simulink model "full_system_nios"  (R2021b)
settings: Solver=FixedStepDiscrete  StartTime=0.0  StopTime=250000  RelTol=1e-3
model workspace (MAT data in the model file):
  out_size = 0
undefined symbols (not defined in the file): betas, bias, DiscIntNeverNeededParam, mus, scale, sigmas
libraries: hdlsllib x2
(part 1 of 3)
settings Model: DataTypeOverride=Off  SimulationMode=accelerator  Creator=local_adm  LastModifiedBy=local_adm
settings SolverCC: AlgebraicLoopSolver=TrustRegion
settings DataIOCC: LimitDataPoints=on  SaveOutput=off  SaveTime=off
settings OptimizationCC: BlockReduction=off  ConditionallyExecuteInputs=off  DefaultParameterBehavior=Inlined  LifeSpan=inf
settings DebuggingCC: AlgebraicLoopMsg=error  SingleTaskRateTransMsg=error  ParameterPrecisionLossMsg=none  AllowSymbolicDim=off  StrictBusMsg=ErrorOnBusTreatedAsVector  SFUnexpectedBacktrackingDiag=warning  SFNoUnconditionalDefaultTransitionDiag=warning  SFExecutionAtInitializationDiag=none  SFMachineParentedDataDiag=warning  ArithmeticOperatorsInVariantConditions=warning
settings HardwareCC: ProdBitPerPointer=32  ProdBitPerSizeT=32  ProdBitPerPtrDiffT=32  ProdLargestAtomicFloat=None  ProdIntDivRoundTo=Undefined  ProdEndianess=Unspecified  ProdWordSize=32  ProdHWDeviceType=ASIC/FPGA->ASIC/FPGA  ProdEqTarget=off
settings SFSimCC: SimUseLocalCustomCode=off  CustomCodeUndefinedFunction=UseInterfaceOnly
settings RTWCC: RTWUseLocalCustomCode=off
settings CodeAppCC: StateflowObjectComments=on
settings GRTTargetCC: TargetLangStandard=C89/C90 (ANSI)
settings ConfigComp: CovScope=ReferencedModels  CovMetricSettings=dw  CovSaveCumulativeToWorkspaceVar=on  CovSaveSingleToWorkspaceVar=on  CovExternalEMLEnable=off  CovSFcnEnable=off

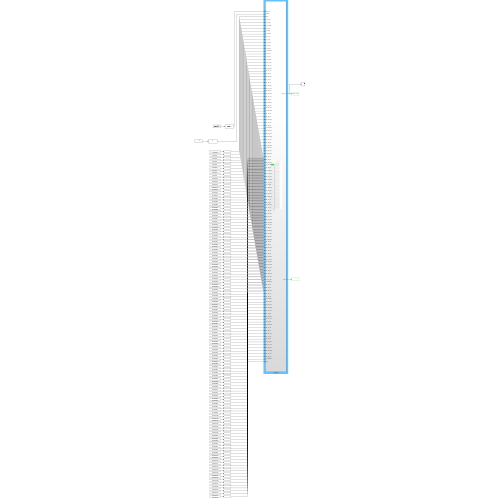
[thumbnail: Simulink's stored preview of the top-level diagram]
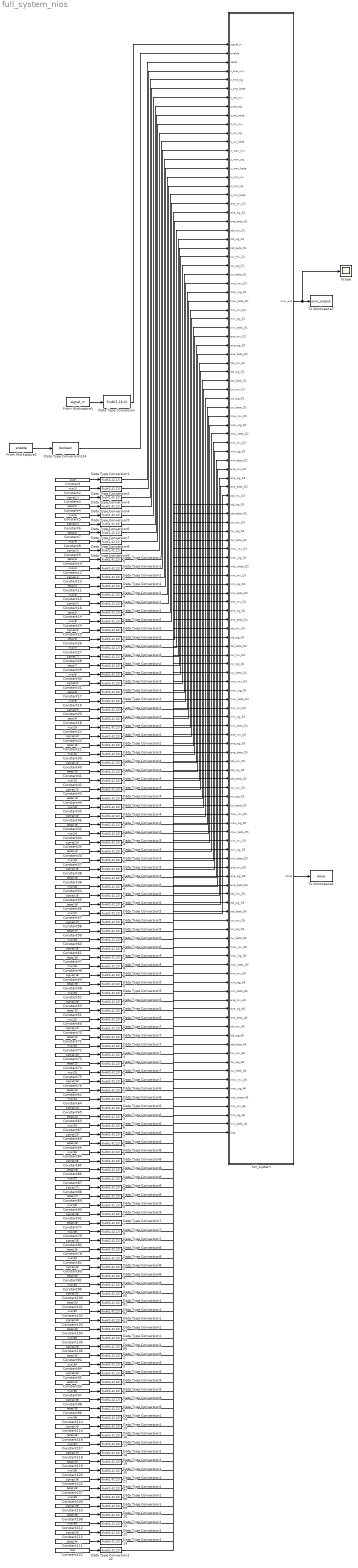
== system full_system_nios ==
  Constant : Constant  Value=scale  VectorParams1D=off  SampleTime=-1
  Constant10 : Constant  Value=betas(3)  VectorParams1D=off  SampleTime=-1
  Constant100 : Constant  Value=sigmas(31)  VectorParams1D=off  SampleTime=-1
  Constant101 : Constant  Value=betas(31)  VectorParams1D=off  SampleTime=-1
  Constant102 : Constant  Value=mus(32)  VectorParams1D=off  SampleTime=-1
  Constant103 : Constant  Value=sigmas(32)  VectorParams1D=off  SampleTime=-1
  Constant104 : Constant  Value=betas(32)  VectorParams1D=off  SampleTime=-1
  Constant105 : Constant  Value=mus(33)  VectorParams1D=off  SampleTime=-1
  Constant106 : Constant  Value=sigmas(33)  VectorParams1D=off  SampleTime=-1
  Constant107 : Constant  Value=betas(38)  VectorParams1D=off  SampleTime=-1
  Constant108 : Constant  Value=betas(39)  VectorParams1D=off  SampleTime=-1
  Constant109 : Constant  Value=mus(39)  VectorParams1D=off  SampleTime=-1
  Constant11 : Constant  Value=betas(4)  VectorParams1D=off  SampleTime=-1
  Constant110 : Constant  Value=sigmas(39)  VectorParams1D=off  SampleTime=-1
  Constant111 : Constant  Value=betas(40)  VectorParams1D=off  SampleTime=-1
  Constant112 : Constant  Value=mus(40)  VectorParams1D=off  SampleTime=-1
  Constant113 : Constant  Value=sigmas(40)  VectorParams1D=off  SampleTime=-1
  Constant114 : Constant  Value=mus(36)  VectorParams1D=off  SampleTime=-1
  Constant115 : Constant  Value=sigmas(36)  VectorParams1D=off  SampleTime=-1
  Constant116 : Constant  Value=betas(36)  VectorParams1D=off  SampleTime=-1
  Constant117 : Constant  Value=mus(37)  VectorParams1D=off  SampleTime=-1
  Constant118 : Constant  Value=sigmas(37)  VectorParams1D=off  SampleTime=-1
  Constant119 : Constant  Value=betas(37)  VectorParams1D=off  SampleTime=-1
  Constant12 : Constant  Value=mus(4)  VectorParams1D=off  SampleTime=-1
  Constant120 : Constant  Value=mus(38)  VectorParams1D=off  SampleTime=-1
  Constant121 : Constant  Value=sigmas(38)  VectorParams1D=off  SampleTime=-1
  Constant122 : Constant  Value=bias  VectorParams1D=off  SampleTime=-1
  Constant13 : Constant  Value=sigmas(4)  VectorParams1D=off  SampleTime=-1
  Constant14 : Constant  Value=betas(5)  VectorParams1D=off  SampleTime=-1
  Constant15 : Constant  Value=mus(5)  VectorParams1D=off  SampleTime=-1
  Constant16 : Constant  Value=sigmas(5)  VectorParams1D=off  SampleTime=-1
  Constant17 : Constant  Value=betas(8)  VectorParams1D=off  SampleTime=-1
  Constant18 : Constant  Value=betas(9)  VectorParams1D=off  SampleTime=-1
  Constant19 : Constant  Value=mus(9)  VectorParams1D=off  SampleTime=-1
  Constant2 : Constant  Value=mus(1)  VectorParams1D=off  SampleTime=-1
  Constant20 : Constant  Value=sigmas(9)  VectorParams1D=off  SampleTime=-1
  Constant21 : Constant  Value=betas(10)  VectorParams1D=off  SampleTime=-1
  Constant22 : Constant  Value=mus(10)  VectorParams1D=off  SampleTime=-1
  Constant23 : Constant  Value=sigmas(10)  VectorParams1D=off  SampleTime=-1
  Constant24 : Constant  Value=mus(6)  VectorParams1D=off  SampleTime=-1
  Constant25 : Constant  Value=sigmas(6)  VectorParams1D=off  SampleTime=-1
  Constant26 : Constant  Value=betas(6)  VectorParams1D=off  SampleTime=-1
  Constant27 : Constant  Value=mus(7)  VectorParams1D=off  SampleTime=-1
  Constant28 : Constant  Value=sigmas(7)  VectorParams1D=off  SampleTime=-1
  Constant29 : Constant  Value=betas(7)  VectorParams1D=off  SampleTime=-1
  Constant3 : Constant  Value=sigmas(1)  VectorParams1D=off  SampleTime=-1
  Constant30 : Constant  Value=mus(8)  VectorParams1D=off  SampleTime=-1
  Constant31 : Constant  Value=sigmas(8)  VectorParams1D=off  SampleTime=-1
  Constant32 : Constant  Value=betas(13)  VectorParams1D=off  SampleTime=-1
  Constant33 : Constant  Value=betas(14)  VectorParams1D=off  SampleTime=-1
  Constant34 : Constant  Value=mus(14)  VectorParams1D=off  SampleTime=-1
  Constant35 : Constant  Value=sigmas(14)  VectorParams1D=off  SampleTime=-1
  Constant36 : Constant  Value=betas(15)  VectorParams1D=off  SampleTime=-1
  Constant37 : Constant  Value=mus(15)  VectorParams1D=off  SampleTime=-1
  Constant38 : Constant  Value=sigmas(15)  VectorParams1D=off  SampleTime=-1
  Constant39 : Constant  Value=mus(11)  VectorParams1D=off  SampleTime=-1
  Constant4 : Constant  Value=betas(1)  VectorParams1D=off  SampleTime=-1
  Constant40 : Constant  Value=sigmas(11)  VectorParams1D=off  SampleTime=-1
  Constant41 : Constant  Value=betas(11)  VectorParams1D=off  SampleTime=-1
  Constant42 : Constant  Value=mus(12)  VectorParams1D=off  SampleTime=-1
  Constant43 : Constant  Value=sigmas(12)  VectorParams1D=off  SampleTime=-1
  Constant44 : Constant  Value=betas(12)  VectorParams1D=off  SampleTime=-1
  Constant45 : Constant  Value=mus(13)  VectorParams1D=off  SampleTime=-1
  Constant46 : Constant  Value=sigmas(13)  VectorParams1D=off  SampleTime=-1
  Constant47 : Constant  Value=betas(18)  VectorParams1D=off  SampleTime=-1
  Constant48 : Constant  Value=betas(19)  VectorParams1D=off  SampleTime=-1
  Constant49 : Constant  Value=mus(19)  VectorParams1D=off  SampleTime=-1
  Constant5 : Constant  Value=mus(2)  VectorParams1D=off  SampleTime=-1
  Constant50 : Constant  Value=sigmas(19)  VectorParams1D=off  SampleTime=-1
  Constant51 : Constant  Value=betas(20)  VectorParams1D=off  SampleTime=-1
  Constant52 : Constant  Value=mus(20)  VectorParams1D=off  SampleTime=-1
  Constant53 : Constant  Value=sigmas(20)  VectorParams1D=off  SampleTime=-1
  Constant54 : Constant  Value=mus(16)  VectorParams1D=off  SampleTime=-1
  Constant55 : Constant  Value=sigmas(16)  VectorParams1D=off  SampleTime=-1
  Constant56 : Constant  Value=betas(16)  VectorParams1D=off  SampleTime=-1
  Constant57 : Constant  Value=mus(17)  VectorParams1D=off  SampleTime=-1
  Constant58 : Constant  Value=sigmas(17)  VectorParams1D=off  SampleTime=-1
  Constant59 : Constant  Value=betas(17)  VectorParams1D=off  SampleTime=-1
  Constant6 : Constant  Value=sigmas(2)  VectorParams1D=off  SampleTime=-1
  Constant60 : Constant  Value=mus(18)  VectorParams1D=off  SampleTime=-1
  Constant61 : Constant  Value=sigmas(18)  VectorParams1D=off  SampleTime=-1
  Constant62 : Constant  Value=betas(23)  VectorParams1D=off  SampleTime=-1
  Constant63 : Constant  Value=betas(24)  VectorParams1D=off  SampleTime=-1
  Constant64 : Constant  Value=mus(24)  VectorParams1D=off  SampleTime=-1
  Constant65 : Constant  Value=sigmas(24)  VectorParams1D=off  SampleTime=-1
  Constant66 : Constant  Value=betas(25)  VectorParams1D=off  SampleTime=-1
  Constant67 : Constant  Value=mus(25)  VectorParams1D=off  SampleTime=-1
  Constant68 : Constant  Value=sigmas(25)  VectorParams1D=off  SampleTime=-1
  Constant69 : Constant  Value=mus(21)  VectorParams1D=off  SampleTime=-1
  Constant7 : Constant  Value=betas(2)  VectorParams1D=off  SampleTime=-1
  Constant70 : Constant  Value=sigmas(21)  VectorParams1D=off  SampleTime=-1
  Constant71 : Constant  Value=betas(21)  VectorParams1D=off  SampleTime=-1
  Constant72 : Constant  Value=mus(22)  VectorParams1D=off  SampleTime=-1
  Constant73 : Constant  Value=sigmas(22)  VectorParams1D=off  SampleTime=-1
  Constant74 : Constant  Value=betas(22)  VectorParams1D=off  SampleTime=-1
  Constant75 : Constant  Value=mus(23)  VectorParams1D=off  SampleTime=-1
  Constant76 : Constant  Value=sigmas(23)  VectorParams1D=off  SampleTime=-1
  Constant77 : Constant  Value=betas(28)  VectorParams1D=off  SampleTime=-1
  Constant78 : Constant  Value=betas(29)  VectorParams1D=off  SampleTime=-1
  Constant79 : Constant  Value=mus(29)  VectorParams1D=off  SampleTime=-1
  Constant8 : Constant  Value=mus(3)  VectorParams1D=off  SampleTime=-1
  Constant80 : Constant  Value=sigmas(29)  VectorParams1D=off  SampleTime=-1
  Constant81 : Constant  Value=betas(30)  VectorParams1D=off  SampleTime=-1
  Constant82 : Constant  Value=mus(30)  VectorParams1D=off  SampleTime=-1
  Constant83 : Constant  Value=sigmas(30)  VectorParams1D=off  SampleTime=-1
  Constant84 : Constant  Value=mus(26)  VectorParams1D=off  SampleTime=-1
  Constant85 : Constant  Value=sigmas(26)  VectorParams1D=off  SampleTime=-1
  Constant86 : Constant  Value=betas(26)  VectorParams1D=off  SampleTime=-1
  Constant87 : Constant  Value=mus(27)  VectorParams1D=off  SampleTime=-1
  Constant88 : Constant  Value=sigmas(27)  VectorParams1D=off  SampleTime=-1
  Constant89 : Constant  Value=betas(27)  VectorParams1D=off  SampleTime=-1
  Constant9 : Constant  Value=sigmas(3)  VectorParams1D=off  SampleTime=-1
  Constant90 : Constant  Value=mus(28)  VectorParams1D=off  SampleTime=-1
  Constant91 : Constant  Value=sigmas(28)  VectorParams1D=off  SampleTime=-1
  Constant92 : Constant  Value=betas(33)  VectorParams1D=off  SampleTime=-1
  Constant93 : Constant  Value=betas(34)  VectorParams1D=off  SampleTime=-1
  Constant94 : Constant  Value=mus(34)  VectorParams1D=off  SampleTime=-1
  Constant95 : Constant  Value=sigmas(34)  VectorParams1D=off  SampleTime=-1
  Constant96 : Constant  Value=betas(35)  VectorParams1D=off  SampleTime=-1
  Constant97 : Constant  Value=mus(35)  VectorParams1D=off  SampleTime=-1
  Constant98 : Constant  Value=sigmas(35)  VectorParams1D=off  SampleTime=-1
  Constant99 : Constant  Value=mus(31)  VectorParams1D=off  SampleTime=-1
  Data Type Conversion : DataTypeConversion  OutMax=2  OutDataTypeStr=fixdt(1,16,4)
  Data Type Conversion{1..122} (122 alike) : DataTypeConversion  OutMax=2  OutDataTypeStr=fixdt(1,42,12)
  Data Type Conversion124 : DataTypeConversion  OutMax=1  OutDataTypeStr=boolean
  From Workspace1 : FromWorkspace  VariableName=signal_in  SampleTime=1  OutputAfterFinalValue=Setting to zero
  From Workspace2 : FromWorkspace  VariableName=enable  SampleTime=1  OutputAfterFinalValue=Setting to zero
  Scope : Scope
  To Workspace1 : ToWorkspace  VariableName=done  SampleTime=-1
  To Workspace7 : ToWorkspace  VariableName=svm_output  SampleTime=-1
  full_system : Subsystem
  wires:
  From Workspace1/1 -> Data Type Conversion/1
  Constant/1 -> Data Type Conversion1/1
  Constant2/1 -> Data Type Conversion2/1
  Constant3/1 -> Data Type Conversion3/1
  Constant4/1 -> Data Type Conversion4/1
  Constant5/1 -> Data Type Conversion5/1
  Constant6/1 -> Data Type Conversion6/1
  Constant7/1 -> Data Type Conversion7/1
  Constant9/1 -> Data Type Conversion9/1
  Constant8/1 -> Data Type Conversion8/1
  Constant13/1 -> Data Type Conversion12/1
  Constant12/1 -> Data Type Conversion11/1
  Constant11/1 -> Data Type Conversion13/1
  Constant10/1 -> Data Type Conversion10/1
  Constant14/1 -> Data Type Conversion16/1
  Constant16/1 -> Data Type Conversion15/1
  Constant15/1 -> Data Type Conversion14/1
  Constant21/1 -> Data Type Conversion23/1
  Constant25/1 -> Data Type Conversion25/1
  Constant31/1 -> Data Type Conversion31/1
  Constant30/1 -> Data Type Conversion30/1
  Constant24/1 -> Data Type Conversion24/1
  Constant28/1 -> Data Type Conversion28/1
  Constant20/1 -> Data Type Conversion19/1
  Constant17/1 -> Data Type Conversion17/1
  Constant27/1 -> Data Type Conversion27/1
  Constant18/1 -> Data Type Conversion20/1
  Constant19/1 -> Data Type Conversion18/1
  Constant29/1 -> Data Type Conversion29/1
  Constant26/1 -> Data Type Conversion26/1
  Constant22/1 -> Data Type Conversion21/1
  Constant23/1 -> Data Type Conversion22/1
  Constant36/1 -> Data Type Conversion38/1
  Constant40/1 -> Data Type Conversion40/1
  Constant46/1 -> Data Type Conversion46/1
  Constant45/1 -> Data Type Conversion45/1
  Constant39/1 -> Data Type Conversion39/1
  Constant43/1 -> Data Type Conversion43/1
  Constant35/1 -> Data Type Conversion34/1
  Constant32/1 -> Data Type Conversion32/1
  Constant42/1 -> Data Type Conversion42/1
  Constant33/1 -> Data Type Conversion35/1
  Constant34/1 -> Data Type Conversion33/1
  Constant44/1 -> Data Type Conversion44/1
  Constant41/1 -> Data Type Conversion41/1
  Constant37/1 -> Data Type Conversion36/1
  Constant38/1 -> Data Type Conversion37/1
  Constant51/1 -> Data Type Conversion53/1
  Constant55/1 -> Data Type Conversion55/1
  Constant61/1 -> Data Type Conversion61/1
  Constant60/1 -> Data Type Conversion60/1
  Constant54/1 -> Data Type Conversion54/1
  Constant58/1 -> Data Type Conversion58/1
  Constant50/1 -> Data Type Conversion49/1
  Constant47/1 -> Data Type Conversion47/1
  Constant57/1 -> Data Type Conversion57/1
  Constant48/1 -> Data Type Conversion50/1
  Constant49/1 -> Data Type Conversion48/1
  Constant59/1 -> Data Type Conversion59/1
  Constant56/1 -> Data Type Conversion56/1
  Constant52/1 -> Data Type Conversion51/1
  Constant53/1 -> Data Type Conversion52/1
  Constant66/1 -> Data Type Conversion68/1
  Constant70/1 -> Data Type Conversion70/1
  Constant76/1 -> Data Type Conversion76/1
  Constant75/1 -> Data Type Conversion75/1
  Constant69/1 -> Data Type Conversion69/1
  Constant73/1 -> Data Type Conversion73/1
  Constant65/1 -> Data Type Conversion64/1
  Constant62/1 -> Data Type Conversion62/1
  Constant72/1 -> Data Type Conversion72/1
  Constant63/1 -> Data Type Conversion65/1
  Constant64/1 -> Data Type Conversion63/1
  Constant74/1 -> Data Type Conversion74/1
  Constant71/1 -> Data Type Conversion71/1
  Constant67/1 -> Data Type Conversion66/1
  Constant68/1 -> Data Type Conversion67/1
  Constant81/1 -> Data Type Conversion83/1
  Constant85/1 -> Data Type Conversion85/1
  Constant91/1 -> Data Type Conversion91/1
  Constant90/1 -> Data Type Conversion90/1
  Constant84/1 -> Data Type Conversion84/1
  Constant88/1 -> Data Type Conversion88/1
  Constant80/1 -> Data Type Conversion79/1
  Constant77/1 -> Data Type Conversion77/1
  Constant87/1 -> Data Type Conversion87/1
  Constant78/1 -> Data Type Conversion80/1
  Constant79/1 -> Data Type Conversion78/1
  Constant89/1 -> Data Type Conversion89/1
  Constant86/1 -> Data Type Conversion86/1
  Constant82/1 -> Data Type Conversion81/1
  Constant83/1 -> Data Type Conversion82/1
  Constant96/1 -> Data Type Conversion98/1
  Constant100/1 -> Data Type Conversion100/1
  Constant106/1 -> Data Type Conversion106/1
  Constant105/1 -> Data Type Conversion105/1
  Constant99/1 -> Data Type Conversion99/1
  Constant103/1 -> Data Type Conversion103/1
  Constant95/1 -> Data Type Conversion94/1
  Constant92/1 -> Data Type Conversion92/1
  Constant102/1 -> Data Type Conversion102/1
  Constant93/1 -> Data Type Conversion95/1
  Constant94/1 -> Data Type Conversion93/1
  Constant104/1 -> Data Type Conversion104/1
  Constant101/1 -> Data Type Conversion101/1
  Constant97/1 -> Data Type Conversion96/1
  Constant98/1 -> Data Type Conversion97/1
  Constant111/1 -> Data Type Conversion113/1
  Constant115/1 -> Data Type Conversion115/1
  Constant121/1 -> Data Type Conversion121/1
  Constant120/1 -> Data Type Conversion120/1
  Constant114/1 -> Data Type Conversion114/1
  Constant118/1 -> Data Type Conversion118/1
  Constant110/1 -> Data Type Conversion109/1
  Constant107/1 -> Data Type Conversion107/1
  Constant117/1 -> Data Type Conversion117/1
  Constant108/1 -> Data Type Conversion110/1
  Constant109/1 -> Data Type Conversion108/1
  Constant119/1 -> Data Type Conversion119/1
  Constant116/1 -> Data Type Conversion116/1
  Constant112/1 -> Data Type Conversion111/1
  Constant113/1 -> Data Type Conversion112/1
  Constant122/1 -> Data Type Conversion122/1
  Data Type Conversion/1 -> full_system/1(signal_in)
  Data Type Conversion124/1 -> full_system/2(enable)
  Data Type Conversion1/1 -> full_system/3(scale)
  Data Type Conversion2/1 -> full_system/4(s_ene_mu)
  Data Type Conversion3/1 -> full_system/5(s_ene_sig)
  Data Type Conversion4/1 -> full_system/6(s_ene_beta)
  Data Type Conversion5/1 -> full_system/7(s_act_mu)
  Data Type Conversion6/1 -> full_system/8(s_act_sig)
  Data Type Conversion7/1 -> full_system/9(s_act_beta)
  Data Type Conversion8/1 -> full_system/10(s_cur_mu)
  Data Type Conversion9/1 -> full_system/11(s_cur_sig)
  Data Type Conversion10/1 -> full_system/12(s_cur_beta)
  Data Type Conversion11/1 -> full_system/13(s_max_mu)
  Data Type Conversion12/1 -> full_system/14(s_max_sig)
  Data Type Conversion13/1 -> full_system/15(s_max_beta)
  Data Type Conversion14/1 -> full_system/16(s_min_mu)
  Data Type Conversion15/1 -> full_system/17(s_min_sig)
  Data Type Conversion16/1 -> full_system/18(s_min_beta)
  Data Type Conversion24/1 -> full_system/19(ene_mu_D1)
  Data Type Conversion25/1 -> full_system/20(ene_sig_D1)
  Data Type Conversion26/1 -> full_system/21(ene_beta_D1)
  Data Type Conversion27/1 -> full_system/22(std_mu_D1)
  Data Type Conversion28/1 -> full_system/23(std_sig_D1)
  Data Type Conversion29/1 -> full_system/24(std_beta_D1)
  Data Type Conversion30/1 -> full_system/25(cur_mu_D1)
  Data Type Conversion31/1 -> full_system/26(cur_sig_D1)
  Data Type Conversion17/1 -> full_system/27(cur_beta_D1)
  Data Type Conversion18/1 -> full_system/28(max_mu_D1)
  Data Type Conversion19/1 -> full_system/29(max_sig_D1)
  Data Type Conversion20/1 -> full_system/30(max_beta_D1)
  Data Type Conversion21/1 -> full_system/31(min_mu_D1)
  Data Type Conversion22/1 -> full_system/32(min_sig_D1)
  Data Type Conversion23/1 -> full_system/33(min_beta_D1)
  Data Type Conversion39/1 -> full_system/34(ene_mu_D2)
  Data Type Conversion40/1 -> full_system/35(ene_sig_D2)
  Data Type Conversion41/1 -> full_system/36(ene_beta_D2)
  Data Type Conversion42/1 -> full_system/37(std_mu_D2)
  Data Type Conversion43/1 -> full_system/38(std_sig_D2)
  Data Type Conversion44/1 -> full_system/39(std_beta_D2)
  Data Type Conversion45/1 -> full_system/40(cur_mu_D2)
  Data Type Conversion46/1 -> full_system/41(cur_sig_D2)
  Data Type Conversion32/1 -> full_system/42(cur_beta_D2)
  Data Type Conversion33/1 -> full_system/43(max_mu_D2)
  Data Type Conversion34/1 -> full_system/44(max_sig_D2)
  Data Type Conversion35/1 -> full_system/45(max_beta_D2)
  Data Type Conversion36/1 -> full_system/46(min_mu_D2)
  Data Type Conversion37/1 -> full_system/47(min_sig_D2)
  Data Type Conversion38/1 -> full_system/48(min_beta_D2)
  Data Type Conversion54/1 -> full_system/49(ene_mu_D3)
  Data Type Conversion55/1 -> full_system/50(ene_sig_D3)
  Data Type Conversion56/1 -> full_system/51(ene_beta_D3)
  Data Type Conversion57/1 -> full_system/52(std_mu_D3)
  Data Type Conversion58/1 -> full_system/53(std_sig_D3)
  Data Type Conversion59/1 -> full_system/54(std_beta_D3)
  Data Type Conversion60/1 -> full_system/55(cur_mu_D3)
  Data Type Conversion61/1 -> full_system/56(cur_sig_D3)
  Data Type Conversion47/1 -> full_system/57(cur_beta_D3)
  Data Type Conversion48/1 -> full_system/58(max_mu_D3)
  Data Type Conversion49/1 -> full_system/59(max_sig_D3)
  Data Type Conversion50/1 -> full_system/60(max_beta_D3)
  Data Type Conversion51/1 -> full_system/61(min_mu_D3)
  Data Type Conversion52/1 -> full_system/62(min_sig_D3)
  Data Type Conversion53/1 -> full_system/63(min_beta_D3)
  Data Type Conversion69/1 -> full_system/64(ene_mu_D4)
  Data Type Conversion70/1 -> full_system/65(ene_sig_D4)
  Data Type Conversion71/1 -> full_system/66(ene_beta_D4)
  Data Type Conversion72/1 -> full_system/67(std_mu_D4)
  Data Type Conversion73/1 -> full_system/68(std_sig_D4)
  Data Type Conversion74/1 -> full_system/69(std_beta_D4)
  Data Type Conversion75/1 -> full_system/70(cur_mu_D4)
  Data Type Conversion76/1 -> full_system/71(cur_sig_D4)
  Data Type Conversion62/1 -> full_system/72(cur_beta_D4)
  Data Type Conversion63/1 -> full_system/73(max_mu_D4)
  Data Type Conversion64/1 -> full_system/74(max_sig_D4)
  Data Type Conversion65/1 -> full_system/75(max_beta_D4)
  Data Type Conversion66/1 -> full_system/76(min_mu_D4)
  Data Type Conversion67/1 -> full_system/77(min_sig_D4)
  Data Type Conversion68/1 -> full_system/78(min_beta_D4)
  Data Type Conversion84/1 -> full_system/79(ene_mu_D5)
  Data Type Conversion85/1 -> full_system/80(ene_sig_D5)
  Data Type Conversion86/1 -> full_system/81(ene_beta_D5)
  Data Type Conversion87/1 -> full_system/82(std_mu_D5)
  Data Type Conversion88/1 -> full_system/83(std_sig_D5)
  Data Type Conversion89/1 -> full_system/84(std_beta_D5)
  Data Type Conversion90/1 -> full_system/85(cur_mu_D5)
  Data Type Conversion91/1 -> full_system/86(cur_sig_D5)
  Data Type Conversion77/1 -> full_system/87(cur_beta_D5)
  Data Type Conversion78/1 -> full_system/88(max_mu_D5)
  Data Type Conversion79/1 -> full_system/89(max_sig_D5)
  Data Type Conversion80/1 -> full_system/90(max_beta_D5)
  Data Type Conversion81/1 -> full_system/91(min_mu_D5)
  Data Type Conversion82/1 -> full_system/92(min_sig_D5)
  Data Type Conversion83/1 -> full_system/93(min_beta_D5)
  Data Type Conversion99/1 -> full_system/94(ene_mu_D6)
  Data Type Conversion100/1 -> full_system/95(ene_sig_D6)
  Data Type Conversion101/1 -> full_system/96(ene_beta_D6)
  Data Type Conversion102/1 -> full_system/97(std_mu_D6)
  Data Type Conversion103/1 -> full_system/98(std_sig_D6)
  Data Type Conversion104/1 -> full_system/99(std_beta_D6)
  Data Type Conversion105/1 -> full_system/100(cur_mu_D6)
  Data Type Conversion106/1 -> full_system/101(cur_sig_D6)
  Data Type Conversion92/1 -> full_system/102(cur_beta_D6)
  Data Type Conversion93/1 -> full_system/103(max_mu_D6)
  Data Type Conversion94/1 -> full_system/104(max_sig_D6)
  Data Type Conversion95/1 -> full_system/105(max_beta_D6)
  Data Type Conversion96/1 -> full_system/106(min_mu_D6)
  Data Type Conversion97/1 -> full_system/107(min_sig_D6)
  Data Type Conversion98/1 -> full_system/108(min_beta_D6)
  Data Type Conversion114/1 -> full_system/109(ene_mu_A6)
  Data Type Conversion115/1 -> full_system/110(ene_sig_A6)
  Data Type Conversion116/1 -> full_system/111(ene_beta_A6)
  Data Type Conversion117/1 -> full_system/112(std_mu_A6)
  Data Type Conversion118/1 -> full_system/113(std_sig_A6)
  Data Type Conversion119/1 -> full_system/114(std_beta_A6)
  Data Type Conversion120/1 -> full_system/115(cur_mu_A6)
  Data Type Conversion121/1 -> full_system/116(cur_sig_A6)
  Data Type Conversion107/1 -> full_system/117(cur_beta_A6)
  Data Type Conversion108/1 -> full_system/118(max_mu_A6)
  Data Type Conversion109/1 -> full_system/119(max_sig_A6)
  Data Type Conversion110/1 -> full_system/120(max_beta_A6)
  Data Type Conversion111/1 -> full_system/121(min_mu_A6)
  Data Type Conversion112/1 -> full_system/122(min_sig_A6)
  Data Type Conversion113/1 -> full_system/123(min_beta_A6)
  Data Type Conversion122/1 -> full_system/124(bias)
  full_system/1(svm_out) -> Scope/1, To Workspace7/1
  From Workspace2/1 -> Data Type Conversion124/1
  full_system/2(done) -> To Workspace1/1

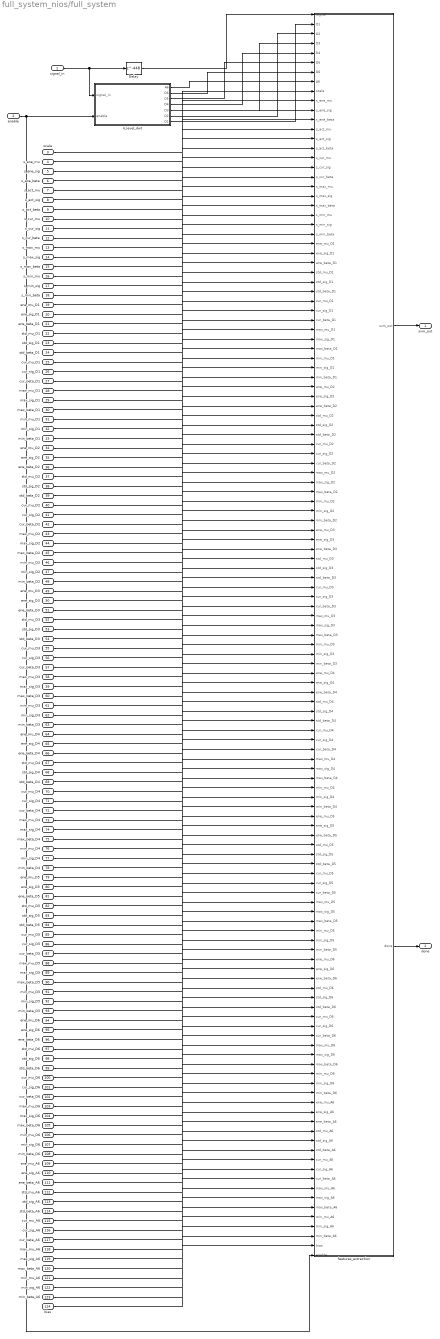
== system full_system_nios/full_system ==
  signal_in : Inport
  enable : Inport  Port=2
  scale : Inport  Port=3
  s_ene_mu : Inport  Port=4
  s_ene_sig : Inport  Port=5
  s_ene_beta : Inport  Port=6
  s_act_mu : Inport  Port=7
  s_act_sig : Inport  Port=8
  s_act_beta : Inport  Port=9
  s_cur_mu : Inport  Port=10
  s_cur_sig : Inport  Port=11
  s_cur_beta : Inport  Port=12
  s_max_mu : Inport  Port=13
  s_max_sig : Inport  Port=14
  s_max_beta : Inport  Port=15
  s_min_mu : Inport  Port=16
  s_min_sig : Inport  Port=17
  s_min_beta : Inport  Port=18
  ene_mu_D1 : Inport  Port=19
  ene_sig_D1 : Inport  Port=20
  ene_beta_D1 : Inport  Port=21
  std_mu_D1 : Inport  Port=22
  std_sig_D1 : Inport  Port=23
  std_beta_D1 : Inport  Port=24
  cur_mu_D1 : Inport  Port=25
  cur_sig_D1 : Inport  Port=26
  cur_beta_D1 : Inport  Port=27
  max_mu_D1 : Inport  Port=28
  max_sig_D1 : Inport  Port=29
  max_beta_D1 : Inport  Port=30
  min_mu_D1 : Inport  Port=31
  min_sig_D1 : Inport  Port=32
  min_beta_D1 : Inport  Port=33
  ene_mu_D2 : Inport  Port=34
  ene_sig_D2 : Inport  Port=35
  ene_beta_D2 : Inport  Port=36
  std_mu_D2 : Inport  Port=37
  std_sig_D2 : Inport  Port=38
  std_beta_D2 : Inport  Port=39
  cur_mu_D2 : Inport  Port=40
  cur_sig_D2 : Inport  Port=41
  cur_beta_D2 : Inport  Port=42
  max_mu_D2 : Inport  Port=43
  max_sig_D2 : Inport  Port=44
  max_beta_D2 : Inport  Port=45
  min_mu_D2 : Inport  Port=46
  min_sig_D2 : Inport  Port=47
  min_beta_D2 : Inport  Port=48
  ene_mu_D3 : Inport  Port=49
  ene_sig_D3 : Inport  Port=50
  ene_beta_D3 : Inport  Port=51
  std_mu_D3 : Inport  Port=52
  std_sig_D3 : Inport  Port=53
  std_beta_D3 : Inport  Port=54
  cur_mu_D3 : Inport  Port=55
  cur_sig_D3 : Inport  Port=56
  cur_beta_D3 : Inport  Port=57
  max_mu_D3 : Inport  Port=58
  max_sig_D3 : Inport  Port=59
  max_beta_D3 : Inport  Port=60
  min_mu_D3 : Inport  Port=61
  min_sig_D3 : Inport  Port=62
  min_beta_D3 : Inport  Port=63
  ene_mu_D4 : Inport  Port=64
  ene_sig_D4 : Inport  Port=65
  ene_beta_D4 : Inport  Port=66
  std_mu_D4 : Inport  Port=67
  std_sig_D4 : Inport  Port=68
  std_beta_D4 : Inport  Port=69
  cur_mu_D4 : Inport  Port=70
  cur_sig_D4 : Inport  Port=71
  cur_beta_D4 : Inport  Port=72
  max_mu_D4 : Inport  Port=73
  max_sig_D4 : Inport  Port=74
  max_beta_D4 : Inport  Port=75
  min_mu_D4 : Inport  Port=76
  min_sig_D4 : Inport  Port=77
  min_beta_D4 : Inport  Port=78
  ene_mu_D5 : Inport  Port=79
  ene_sig_D5 : Inport  Port=80
  ene_beta_D5 : Inport  Port=81
  std_mu_D5 : Inport  Port=82
  std_sig_D5 : Inport  Port=83
  std_beta_D5 : Inport  Port=84
  cur_mu_D5 : Inport  Port=85
  cur_sig_D5 : Inport  Port=86
  cur_beta_D5 : Inport  Port=87
  max_mu_D5 : Inport  Port=88
  max_sig_D5 : Inport  Port=89
  max_beta_D5 : Inport  Port=90
  min_mu_D5 : Inport  Port=91
  min_sig_D5 : Inport  Port=92
  min_beta_D5 : Inport  Port=93
  ene_mu_D6 : Inport  Port=94
  ene_sig_D6 : Inport  Port=95
  ene_beta_D6 : Inport  Port=96
  std_mu_D6 : Inport  Port=97
  std_sig_D6 : Inport  Port=98
  std_beta_D6 : Inport  Port=99
  cur_mu_D6 : Inport  Port=100
  cur_sig_D6 : Inport  Port=101
  cur_beta_D6 : Inport  Port=102
  max_mu_D6 : Inport  Port=103
  max_sig_D6 : Inport  Port=104
  max_beta_D6 : Inport  Port=105
  min_mu_D6 : Inport  Port=106
  min_sig_D6 : Inport  Port=107
  min_beta_D6 : Inport  Port=108
  ene_mu_A6 : Inport  Port=109
  ene_sig_A6 : Inport  Port=110
  ene_beta_A6 : Inport  Port=111
  std_mu_A6 : Inport  Port=112
  std_sig_A6 : Inport  Port=113
  std_beta_A6 : Inport  Port=114
  cur_mu_A6 : Inport  Port=115
  cur_sig_A6 : Inport  Port=116
  cur_beta_A6 : Inport  Port=117
  max_mu_A6 : Inport  Port=118
  max_sig_A6 : Inport  Port=119
  max_beta_A6 : Inport  Port=120
  min_mu_A6 : Inport  Port=121
  min_sig_A6 : Inport  Port=122
  min_beta_A6 : Inport  Port=123
  bias : Inport  Port=124
  4_level_dwt : Subsystem
  Delay : Delay  DelayLength=448  InitialCondition=0  UseCircularBuffer=on
  features_extraction : Subsystem
  svm_out : Outport
  done : Outport  Port=2
  wires:
  max_sig_D5/1 -> features_extraction/95(max_sig_D5)
  4_level_dwt/7(D1) -> features_extraction/2(D1)
  4_level_dwt/4(D4) -> features_extraction/5(D4)
  max_sig_D2/1 -> features_extraction/50(max_sig_D2)
  cur_beta_D1/1 -> features_extraction/33(cur_beta_D1)
  s_cur_sig/1 -> features_extraction/17(s_cur_sig)
  max_sig_D1/1 -> features_extraction/35(max_sig_D1)
  ene_sig_D3/1 -> features_extraction/56(ene_sig_D3)
  4_level_dwt/2(D6) -> features_extraction/7(D6)
  4_level_dwt/5(D3) -> features_extraction/4(D3)
  ene_mu_D5/1 -> features_extraction/85(ene_mu_D5)
  signal_in/1 -> 4_level_dwt/1(signal_in), Delay/1
  min_beta_D3/1 -> features_extraction/69(min_beta_D3)
  max_beta_D4/1 -> features_extraction/81(max_beta_D4)
  max_mu_D4/1 -> features_extraction/79(max_mu_D4)
  std_sig_D2/1 -> features_extraction/44(std_sig_D2)
  4_level_dwt/6(D2) -> features_extraction/3(D2)
  min_beta_A6/1 -> features_extraction/129(min_beta_A6)
  cur_sig_D1/1 -> features_extraction/32(cur_sig_D1)
  Delay/1 -> features_extraction/1(Signal)
  ene_beta_D2/1 -> features_extraction/42(ene_beta_D2)
  std_beta_D5/1 -> features_extraction/90(std_beta_D5)
  std_mu_D2/1 -> features_extraction/43(std_mu_D2)
  std_sig_D3/1 -> features_extraction/59(std_sig_D3)
  4_level_dwt/1(A6) -> features_extraction/8(A6)
  4_level_dwt/3(D5) -> features_extraction/6(D5)
  min_beta_D6/1 -> features_extraction/114(min_beta_D6)
  std_sig_D6/1 -> features_extraction/104(std_sig_D6)
  s_ene_beta/1 -> features_extraction/12(s_ene_beta)
  std_mu_D6/1 -> features_extraction/103(std_mu_D6)
  cur_sig_D4/1 -> features_extraction/77(cur_sig_D4)
  std_sig_D5/1 -> features_extraction/89(std_sig_D5)
  max_mu_D3/1 -> features_extraction/64(max_mu_D3)
  s_max_beta/1 -> features_extraction/21(s_max_beta)
  s_ene_sig/1 -> features_extraction/11(s_ene_sig)
  ene_beta_A6/1 -> features_extraction/117(ene_beta_A6)
  max_sig_D4/1 -> features_extraction/80(max_sig_D4)
  s_act_mu/1 -> features_extraction/13(s_act_mu)
  min_mu_A6/1 -> features_extraction/127(min_mu_A6)
  cur_sig_D2/1 -> features_extraction/47(cur_sig_D2)
  max_beta_D5/1 -> features_extraction/96(max_beta_D5)
  ene_beta_D5/1 -> features_extraction/87(ene_beta_D5)
  ene_beta_D1/1 -> features_extraction/27(ene_beta_D1)
  std_mu_D5/1 -> features_extraction/88(std_mu_D5)
  cur_mu_D3/1 -> features_extraction/61(cur_mu_D3)
  ene_beta_D4/1 -> features_extraction/72(ene_beta_D4)
  cur_sig_D5/1 -> features_extraction/92(cur_sig_D5)
  max_mu_A6/1 -> features_extraction/124(max_mu_A6)
  std_beta_D3/1 -> features_extraction/60(std_beta_D3)
  s_act_sig/1 -> features_extraction/14(s_act_sig)
  s_min_mu/1 -> features_extraction/22(s_min_mu)
  scale/1 -> features_extraction/9(scale)
  s_act_beta/1 -> features_extraction/15(s_act_beta)
  max_sig_D6/1 -> features_extraction/110(max_sig_D6)
  std_beta_D4/1 -> features_extraction/75(std_beta_D4)
  ene_mu_D1/1 -> features_extraction/25(ene_mu_D1)
  cur_mu_D6/1 -> features_extraction/106(cur_mu_D6)
  enable/1 -> 4_level_dwt/2(enable), features_extraction/131(enable)
  cur_mu_A6/1 -> features_extraction/121(cur_mu_A6)
  ene_sig_D5/1 -> features_extraction/86(ene_sig_D5)
  min_sig_D6/1 -> features_extraction/113(min_sig_D6)
  max_beta_D6/1 -> features_extraction/111(max_beta_D6)
  max_mu_D6/1 -> features_extraction/109(max_mu_D6)
  std_sig_D4/1 -> features_extraction/74(std_sig_D4)
  cur_mu_D4/1 -> features_extraction/76(cur_mu_D4)
  ene_mu_D6/1 -> features_extraction/100(ene_mu_D6)
  min_mu_D5/1 -> features_extraction/97(min_mu_D5)
  std_sig_D1/1 -> features_extraction/29(std_sig_D1)
  min_mu_D6/1 -> features_extraction/112(min_mu_D6)
  std_beta_D1/1 -> features_extraction/30(std_beta_D1)
  cur_beta_D5/1 -> features_extraction/93(cur_beta_D5)
  min_sig_A6/1 -> features_extraction/128(min_sig_A6)
  s_min_beta/1 -> features_extraction/24(s_min_beta)
  max_mu_D5/1 -> features_extraction/94(max_mu_D5)
  max_beta_A6/1 -> features_extraction/126(max_beta_A6)
  max_sig_A6/1 -> features_extraction/125(max_sig_A6)
  cur_beta_D6/1 -> features_extraction/108(cur_beta_D6)
  ene_sig_A6/1 -> features_extraction/116(ene_sig_A6)
  ene_mu_D2/1 -> features_extraction/40(ene_mu_D2)
  cur_sig_A6/1 -> features_extraction/122(cur_sig_A6)
  cur_beta_A6/1 -> features_extraction/123(cur_beta_A6)
  cur_sig_D3/1 -> features_extraction/62(cur_sig_D3)
  std_beta_A6/1 -> features_extraction/120(std_beta_A6)
  min_beta_D1/1 -> features_extraction/39(min_beta_D1)
  min_beta_D5/1 -> features_extraction/99(min_beta_D5)
  std_sig_A6/1 -> features_extraction/119(std_sig_A6)
  std_mu_D1/1 -> features_extraction/28(std_mu_D1)
  ene_mu_A6/1 -> features_extraction/115(ene_mu_A6)
  min_sig_D5/1 -> features_extraction/98(min_sig_D5)
  cur_beta_D3/1 -> features_extraction/63(cur_beta_D3)
  bias/1 -> features_extraction/130(bias)
  ene_beta_D6/1 -> features_extraction/102(ene_beta_D6)
  s_cur_beta/1 -> features_extraction/18(s_cur_beta)
  std_mu_A6/1 -> features_extraction/118(std_mu_A6)
  max_mu_D1/1 -> features_extraction/34(max_mu_D1)
  features_extraction/1(svm_out) -> svm_out/1
  min_beta_D4/1 -> features_extraction/84(min_beta_D4)
  std_beta_D6/1 -> features_extraction/105(std_beta_D6)
  cur_beta_D2/1 -> features_extraction/48(cur_beta_D2)
  cur_sig_D6/1 -> features_extraction/107(cur_sig_D6)
  ene_sig_D6/1 -> features_extraction/101(ene_sig_D6)
  cur_mu_D2/1 -> features_extraction/46(cur_mu_D2)
  min_mu_D3/1 -> features_extraction/67(min_mu_D3)
  cur_mu_D5/1 -> features_extraction/91(cur_mu_D5)
  ene_sig_D1/1 -> features_extraction/26(ene_sig_D1)
  min_mu_D4/1 -> features_extraction/82(min_mu_D4)
  s_cur_mu/1 -> features_extraction/16(s_cur_mu)
  ene_sig_D4/1 -> features_extraction/71(ene_sig_D4)
  s_min_sig/1 -> features_extraction/23(s_min_sig)
  s_ene_mu/1 -> features_extraction/10(s_ene_mu)
  min_mu_D1/1 -> features_extraction/37(min_mu_D1)
  s_max_mu/1 -> features_extraction/19(s_max_mu)
  min_sig_D1/1 -> features_extraction/38(min_sig_D1)
  cur_mu_D1/1 -> features_extraction/31(cur_mu_D1)
  ene_sig_D2/1 -> features_extraction/41(ene_sig_D2)
  max_mu_D2/1 -> features_extraction/49(max_mu_D2)
  min_mu_D2/1 -> features_extraction/52(min_mu_D2)
  std_beta_D2/1 -> features_extraction/45(std_beta_D2)
  max_beta_D1/1 -> features_extraction/36(max_beta_D1)
  min_beta_D2/1 -> features_extraction/54(min_beta_D2)
  max_beta_D2/1 -> features_extraction/51(max_beta_D2)
  max_sig_D3/1 -> features_extraction/65(max_sig_D3)
  ene_beta_D3/1 -> features_extraction/57(ene_beta_D3)
  max_beta_D3/1 -> features_extraction/66(max_beta_D3)
  s_max_sig/1 -> features_extraction/20(s_max_sig)
  min_sig_D3/1 -> features_extraction/68(min_sig_D3)
  ene_mu_D3/1 -> features_extraction/55(ene_mu_D3)
  std_mu_D3/1 -> features_extraction/58(std_mu_D3)
  cur_beta_D4/1 -> features_extraction/78(cur_beta_D4)
  min_sig_D2/1 -> features_extraction/53(min_sig_D2)
  min_sig_D4/1 -> features_extraction/83(min_sig_D4)
  std_mu_D4/1 -> features_extraction/73(std_mu_D4)
  ene_mu_D4/1 -> features_extraction/70(ene_mu_D4)
  features_extraction/2(done) -> done/1

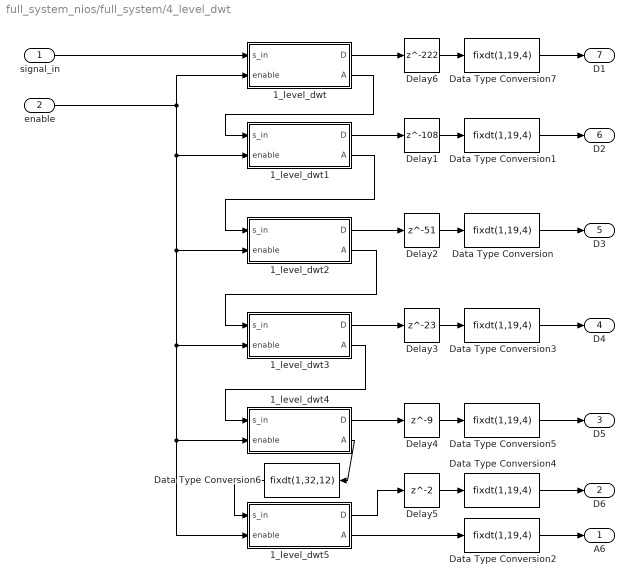
== system full_system_nios/full_system/4_level_dwt ==
  signal_in : Inport
  enable : Inport  Port=2
  1_level_dwt : Subsystem
  1_level_dwt1 : Subsystem
  1_level_dwt2 : Subsystem
  1_level_dwt3 : Subsystem
  1_level_dwt4 : Subsystem
  1_level_dwt5 : Subsystem
  Data Type Conversion{,1..5,7} (7 alike) : DataTypeConversion  OutDataTypeStr=fixdt(1,19,4)
  Data Type Conversion6 : DataTypeConversion  OutDataTypeStr=fixdt(1,32,12)
  Delay1 : Delay  DelayLength=108
  Delay2 : Delay  DelayLength=51
  Delay3 : Delay  DelayLength=23
  Delay4 : Delay  DelayLength=9
  Delay5 : Delay
  Delay6 : Delay  DelayLength=222
  A6 : Outport  VectorParamsAs1DForOutWhenUnconnected=off
  D6 : Outport  Port=2  VectorParamsAs1DForOutWhenUnconnected=off
  D5 : Outport  Port=3  VectorParamsAs1DForOutWhenUnconnected=off
  D4 : Outport  Port=4  VectorParamsAs1DForOutWhenUnconnected=off
  D3 : Outport  Port=5  VectorParamsAs1DForOutWhenUnconnected=off
  D2 : Outport  Port=6  VectorParamsAs1DForOutWhenUnconnected=off
  D1 : Outport  Port=7  VectorParamsAs1DForOutWhenUnconnected=off
  wires:
  signal_in/1 -> 1_level_dwt/1(s_in)
  enable/1 -> 1_level_dwt1/2(enable), 1_level_dwt5/2(enable), 1_level_dwt4/2(enable), 1_level_dwt3/2(enable), 1_level_dwt2/2(enable), 1_level_dwt/2(enable)
  1_level_dwt/2(A) -> 1_level_dwt1/1(s_in)
  1_level_dwt1/2(A) -> 1_level_dwt2/1(s_in)
  1_level_dwt2/2(A) -> 1_level_dwt3/1(s_in)
  1_level_dwt1/1(D) -> Delay1/1
  1_level_dwt2/1(D) -> Delay2/1
  1_level_dwt3/1(D) -> Delay3/1
  Delay2/1 -> Data Type Conversion/1
  Delay1/1 -> Data Type Conversion1/1
  Delay3/1 -> Data Type Conversion3/1
  1_level_dwt3/2(A) -> 1_level_dwt4/1(s_in)
  Delay4/1 -> Data Type Conversion5/1
  1_level_dwt4/1(D) -> Delay4/1
  1_level_dwt5/1(D) -> Delay5/1
  1_level_dwt5/2(A) -> Data Type Conversion2/1
  Delay5/1 -> Data Type Conversion4/1
  Data Type Conversion2/1 -> A6/1
  Data Type Conversion1/1 -> D2/1
  Data Type Conversion/1 -> D3/1
  Data Type Conversion3/1 -> D4/1
  Data Type Conversion4/1 -> D6/1
  Data Type Conversion5/1 -> D5/1
  1_level_dwt4/2(A) -> Data Type Conversion6/1
  Data Type Conversion6/1 -> 1_level_dwt5/1(s_in)
  Delay6/1 -> Data Type Conversion7/1
  1_level_dwt/1(D) -> Delay6/1
  Data Type Conversion7/1 -> D1/1
